simulink model "SYHW_Zscan"  (Simulink 8.1)
settings: Solver=ode5  SolverMode=SingleTasking  StartTime=0.0  StopTime=inf  FixedStep=Ts  RelTol=1e-3
PreLoadFcn:
  | Ts=20e-6;Ts_eHS=8e-7;parameters3;
PostLoadFcn:
  | Ts=20e-6;Ts_eHS=8e-7;parameters3;
InitFcn:
  | Ts=20e-6;Ts_eHS=8e-7;parameters3;
StartFcn:
  | Ts=20e-6;Ts_eHS=8e-7;parameters3;
undefined symbols (not defined in the file or in its folder): Fnom, opsimget, p, SW01
undefined symbols (not defined in the file): LmSI, LrSI, LsSI, RrSI, RsSI
libraries: rtlab x35, rtio_opalrt_common x13, efs_cpuhilios_crtl_lib x4, cpuhilios_lib x4, simulink x3, dspsigops x3, powerlib_extras x1, powerlib_meascontrol x1, rteventslib x1, cpuconverter_lib x1
(part 1 of 2)
settings Model: ARTEMISmethode_block_infos=$$__separator__$$  Creator=Administrator  LastModifiedBy=ncepri  BufferReuse=off
settings DataIOCC: LimitDataPoints=off  SaveFormat=StructureWithTime  SaveOutput=off  SignalLogging=off  DSMLogging=off  SaveTime=off
settings OptimizationCC: BlockReduction=off  OptimizeBlockIOStorage=off  BufferReuse=off  ExpressionFolding=off  LocalBlockOutputs=off
settings DebuggingCC: StrictBusMsg=None
settings GRTTargetCC: CodeReplacementLibrary=None  CPPClassGenCompliant=on
settings ConfigurationSet: Description=SimMechanics 2G

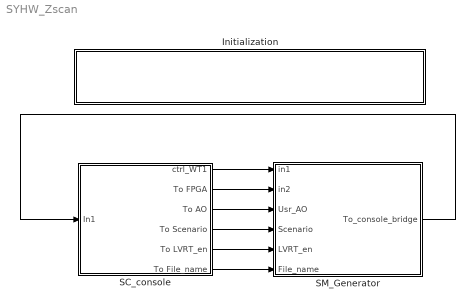
== system SYHW_Zscan ==
  Initialization : Subsystem  mask(Model Functions){InitFcnX=Ts=20e-6;Ts_eHS=8e-7;parameters3;, prel=on, posl=on, inif=on, strf=on}
      mask prompts: InitFcnX "Initialisation"; prel "Preload Function"; posl "PostLoad Function"; inif "InitFcn"; strf "StartFcn"
      mask init:
      | if prel==1
      | 	set_param(bdroot, 'PreLoadFcn', InitFcnX);
      | else
      | 	set_param(bdroot, 'PreLoadFcn', '');
      | end
      | if inif==1
      | 	set_param(bdroot, 'InitFcn', InitFcnX);
      | else
      | 	set_param(bdroot, 'InitFcn', '');
      | end
      | if strf==1
      | 	set_param(bdroot, 'StartFcn', InitFcnX);
      | else
      | 	set_param(bdroot, 'StartFcn', '');
      | end
      | if posl==1
      | 	set_param(bdroot, 'PostLoadFcn', InitFcnX);
      | else
      | 	set_param(bdroot, 'PostLoadFcn', '');
      | end
      | PLF = get_param(bdroot, 'PreLoadFcn');
      | IF = get_param(bdroot, 'InitFcn');
      | SF = get_param(bdroot, 'StartFcn');
      | 
      | 
      | pos = get_param(gcb, 'Position');
      | width = pos(3) - pos(1); height = pos(4) - pos(2);
      mask Display:
      | color('blue')
      | text(5, height*0.25, [ ...
      | upper(bdroot) '\n' ...
      | '- InitFcn. . . . . '  get_param(bdroot, 'InitFcn')  ...
      | ], ...
      | 'horizontalAlignment', 'left', 'verticalAlignment', 'middle') ;
      | text(60,height*0.6,'This is initilization control of the model');
  SC_console : Subsystem
  SM_Generator : Subsystem
  wires:
  SC_console/1(ctrl_WT1) -> SM_Generator/1(in1)
  SM_Generator/1(To_console_bridge) -> SC_console/1(In1)
  SC_console/2(To FPGA) -> SM_Generator/2(in2)
  SC_console/3(To AO) -> SM_Generator/3(Usr_AO)
  SC_console/4(To Scenario) -> SM_Generator/4(Scenario)
  SC_console/5(To LVRT_en) -> SM_Generator/5(LVRT_en)
  SC_console/6(To File_name) -> SM_Generator/6(File_name)

== system SYHW_Zscan/Initialization ==
  Model Info : simulink/Model-Wide Utilities/Model Info  InitialBlockCM=none  BlockCM=None  Frame=on  DisplayStringWithTags=|  HorizontalTextAlignment=Center  LeftAlignmentValue=0.5  SourceBlockDiagram=SYHW_Zscan  TagMaxNumber=20
      | - Version <<<1.0 >>>
      | 
      | - Description :
      | %<Description>
      | 
      | - Created by :     %<Creator>
      | - Creation date : %<Created>
      | - Modified by :    %<ModifiedBy>
      | - Last modif. :   2012.12.11

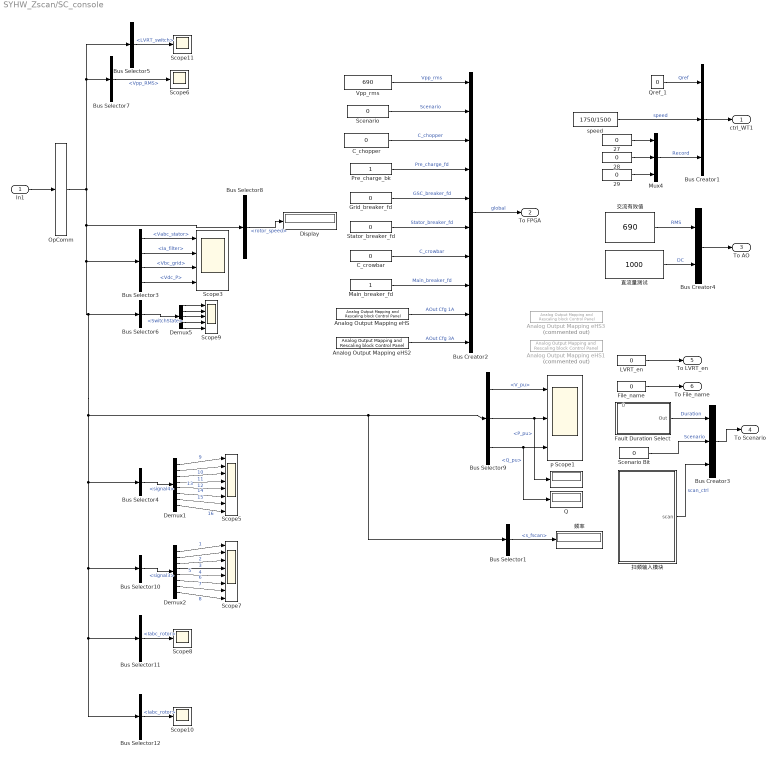
== system SYHW_Zscan/SC_console ==
  note: 0
  In1 : Inport
  " P" : Display
  " Q" : Display
  " 频率" : Display
  27 : Constant  Value=0
  28 : Constant  Value=0
  29 : Constant  Value=0
  Analog Output Mapping eHS : efs_cpuhilios_crtl_lib/Analog Output Mapping and  Rescaling block Control Panel  formFactor=Custom  SigNames={'eHS.Y01' 'eHS.Y02' 'eHS.Y03' 'eHS.Y04' 'eHS.Y05' 'eHS.Y06' 'eHS.Y07' 'eHS.Y08' 'eHS.Y09' 'eHS.Y10' 'eHS.Y11' 'eHS.Y12' 'eHS.Y13' 'eHS.Y14' 'eHS.Y15' 'eHS.Y16' 'eHS.Y17' 'eHS.Y18' 'eHS.Y19' 'eHS.Y20' 'eHS.Y21' 'eHS.Y22' 'eHS.Y23' 'eHS.Y24' 'eHS.Y25' 'eHS.Y26' 'eHS.Y27' 'eHS.Y28' 'eHS.Y29' 'eHS.Y30' 'eHS.Y31' 'eHS.Y32'}  NbUsrAOut=16  signalch0=eHS.Y22  gain0=10/1449  offset0=0  max0=10  min0=-10  signalch1=eHS.Y23  gain1=10/1449  offset1=0  max1=10  min1=-10  signalch2=eHS.Y24  gain2=10/1449  offset2=0  max2=10  min2=-10  signalch3=eHS.Y25  gain3=10/1449  offset3=0  max3=10  min3=-10  signalch4=eHS.Y26  gain4=10/1449  offset4=0  max4=10  min4=-10  signalch5=eHS.Y27  gain5=10/1449  offset5=0  max5=10  min5=-10  signalch6=eHS.Y07  gain6=10/1449  offset6=0  max6=10  min6=-10  signalch7=eHS.Y08  gain7=10/1449  offset7=0  max7=10  min7=-10  signalch8=eHS.Y09  gain8=10/1449  offset8=0  max8=10  min8=-10  signalch9=eHS.Y10  gain9=10/1449  offset9=0  max9=10  min9=-10  signalch10=eHS.Y11  gain10=10/1449  offset10=0  max10=10  min10=-10  signalch11=User16  gain11=0  offset11=0  max11=10  min11=0  signalch12=eHS.Y13  gain12=10/3200*1000/475  offset12=0  max12=10  min12=0  signalch13=User14  gain13=1/160  offset13=0  max13=10  min13=0  signalch14=User15  gain14=1/160  offset14=0  max14=10  min14=0  signalch15=User16  gain15=-10/1600  offset15=0  max15=10  min15=-10  signalch16=User1  gain16=0.0014  offset16=0  max16=5  min16=-5  signalch17=User2  gain17=0.0014  offset17=0  max17=5  min17=-5  signalch18=User3  gain18=0.0014  offset18=0  max18=5  min18=-5  signalch19=User4  gain19=0.00234  offset19=0  max19=5  min19=-5  signalch20=User5  gain20=0.00234  offset20=0  max20=5  min20=-5  signalch21=User6  gain21=0.00234  offset21=0  max21=5  min21=-5  signalch22=User7  gain22=0.00234  offset22=0  max22=5  min22=-5  signalch23=User7  gain23=0.00234  offset23=0  max23=5  min23=-5  signalch24=User9  gain24=0.00174  offset24=0  max24=3  min24=-3  signalch25=User10  gain25=0.000334  offset25=0  max25=3  min25=-3  signalch26=User11  gain26=0.000334  offset26=0  max26=3  min26=-3  signalch27=User12  gain27=0.000334  offset27=0  max27=3  min27=-3  signalch28=User13  gain28=1  offset28=0  max28=16  min28=-16  signalch29=User14  gain29=1  offset29=0  max29=16  min29=-16  signalch30=User15  gain30=1  offset30=0  max30=16  min30=-16  signalch31=User16  gain31=1  offset31=0  max31=16  min31=-16
      link override Display2: Decimation=12500
  Analog Output Mapping eHS1 : efs_cpuhilios_crtl_lib/Analog Output Mapping and  Rescaling block Control Panel  Commented=on  formFactor=Custom  SigNames={'eHS.Y01' 'eHS.Y02' 'eHS.Y03' 'eHS.Y04' 'eHS.Y05' 'eHS.Y06' 'eHS.Y07' 'eHS.Y08' 'eHS.Y09' 'eHS.Y10' 'eHS.Y11' 'eHS.Y12' 'eHS.Y13' 'eHS.Y14' 'eHS.Y15' 'eHS.Y16' 'eHS.Y17' 'eHS.Y18' 'eHS.Y19' 'eHS.Y20' 'eHS.Y21' 'eHS.Y22' 'eHS.Y23' 'eHS.Y24' 'eHS.Y25' 'eHS.Y26' 'eHS.Y27' 'eHS.Y28' 'eHS.Y29' 'eHS.Y30' 'eHS.Y31' 'eHS.Y32'}  NbUsrAOut=16  signalch0=eHS.Y01  gain0=1/240  offset0=0  max0=10  min0=-10  signalch1=eHS.Y02  gain1=1/240  offset1=0  max1=10  min1=-10  signalch2=eHS.Y03  gain2=1/240  offset2=0  max2=10  min2=-10  signalch3=eHS.Y08  gain3=1/722  offset3=0  max3=10  min3=-10  signalch4=eHS.Y09  gain4=1/722  offset4=0  max4=10  min4=-10  signalch5=eHS.Y10  gain5=1/240  offset5=0  max5=10  min5=-10  signalch6=eHS.Y21  gain6=1/240  offset6=0  max6=10  min6=-10  signalch7=eHS.Y22  gain7=1/240  offset7=0  max7=10  min7=-10  signalch8=eHS.Y23  gain8=10/1800*1  offset8=0  max8=10  min8=-10  signalch9=eHS.Y28  gain9=1/100  offset9=0  max9=10  min9=-10  signalch10=eHS.Y29  gain10=1/100  offset10=0  max10=10  min10=-10  signalch11=eHS.Y30  gain11=1/100  offset11=0  max11=14  min11=-14  signalch12=User13  gain12=4/300  offset12=0  max12=4  min12=0  signalch13=User14  gain13=-4/300  offset13=0  max13=5  min13=-5  signalch14=User15  gain14=-4/300  offset14=0  max14=5  min14=-5  signalch15=User16  gain15=4/300  offset15=0  max15=5  min15=0  signalch16=User1  gain16=4/300  offset16=0  max16=3  min16=-3  signalch17=User2  gain17=4/300  offset17=0  max17=4  min17=-4  signalch18=User3  gain18=4/300  offset18=0  max18=4  min18=-4  signalch19=User4  gain19=4/300  offset19=0  max19=4  min19=-4  signalch20=User5  gain20=0.0028427  offset20=0  max20=3  min20=-3  signalch21=User6  gain21=0.0028427  offset21=0  max21=3  min21=-3  signalch22=User7  gain22=0.0028427  offset22=0  max22=3  min22=-3  signalch23=User7  gain23=1  offset23=0  max23=3  min23=-3  signalch24=User9  gain24=1  offset24=0  max24=3  min24=-3  signalch25=User10  gain25=1  offset25=0  max25=16  min25=-16  signalch26=User11  gain26=1  offset26=0  max26=16  min26=-16  signalch27=User12  gain27=1  offset27=0  max27=16  min27=-16  signalch28=User13  gain28=1  offset28=0  max28=16  min28=-16  signalch29=User14  gain29=1  offset29=0  max29=16  min29=-16  signalch30=User15  gain30=1  offset30=0  max30=16  min30=-16  signalch31=User16  gain31=1  offset31=0  max31=16  min31=-16
      link override Display2: Decimation=12500
  Analog Output Mapping eHS2 : efs_cpuhilios_crtl_lib/Analog Output Mapping and  Rescaling block Control Panel  formFactor=Custom  SigNames={'eHS.Y01' 'eHS.Y02' 'eHS.Y03' 'eHS.Y04' 'eHS.Y05' 'eHS.Y06' 'eHS.Y07' 'eHS.Y08' 'eHS.Y09' 'eHS.Y10' 'eHS.Y11' 'eHS.Y12' 'eHS.Y13' 'eHS.Y14' 'eHS.Y15' 'eHS.Y16' 'eHS.Y17' 'eHS.Y18' 'eHS.Y19' 'eHS.Y20' 'eHS.Y21' 'eHS.Y22' 'eHS.Y23' 'eHS.Y24' 'eHS.Y25' 'eHS.Y26' 'eHS.Y27' 'eHS.Y28' 'eHS.Y29' 'eHS.Y30' 'eHS.Y31' 'eHS.Y32'}  NbUsrAOut=16  signalch0=eHS.Y14  gain0=-10/9000*500/330  offset0=0  max0=10  min0=-10  signalch1=eHS.Y15  gain1=-10/9000*500/330  offset1=0  max1=10  min1=-10  signalch2=eHS.Y16  gain2=-10/9000*500/330  offset2=0  max2=10  min2=-10  signalch3=eHS.Y17  gain3=10/10000  offset3=0  max3=10  min3=-10  signalch4=eHS.Y18  gain4=10/10000  offset4=0  max4=10  min4=-10  signalch5=eHS.Y19  gain5=-10/9000*500/330*398/473  offset5=0  max5=10  min5=-10  signalch6=eHS.Y20  gain6=-10/9000*500/330*398/473  offset6=0  max6=10  min6=-10  signalch7=eHS.Y21  gain7=-10/9000*500/330*398/473  offset7=0  max7=10  min7=-10  signalch8=eHS.Y23  gain8=0.00174*500/472*0  offset8=0  max8=3  min8=-3  signalch9=eHS.Y20  gain9=0.000251*353/348*1.315  offset9=0  max9=3  min9=-3  signalch10=eHS.Y21  gain10=0.000251*353/348*1.315  offset10=0  max10=3  min10=-3  signalch11=eHS.Y22  gain11=0.000251*353/348*1.315  offset11=0  max11=3  min11=-3  signalch12=eHS.Y11  gain12=0.00263*0.885*0.864  offset12=0  max12=4  min12=0  signalch13=User14  gain13=0.00263*0.885  offset13=0  max13=5  min13=-5  signalch14=User15  gain14=0.00263*0.885  offset14=0  max14=5  min14=-5  signalch15=User16  gain15=4/300  offset15=0  max15=5  min15=0  signalch16=User1  gain16=4/300  offset16=0  max16=3  min16=-3  signalch17=User2  gain17=4/300  offset17=0  max17=4  min17=-4  signalch18=User3  gain18=4/300  offset18=0  max18=4  min18=-4  signalch19=User4  gain19=4/300  offset19=0  max19=4  min19=-4  signalch20=User5  gain20=0.0028427  offset20=0  max20=3  min20=-3  signalch21=User6  gain21=0.0028427  offset21=0  max21=3  min21=-3  signalch22=User7  gain22=0.0028427  offset22=0  max22=3  min22=-3  signalch23=User7  gain23=1  offset23=0  max23=3  min23=-3  signalch24=User9  gain24=1  offset24=0  max24=3  min24=-3  signalch25=User10  gain25=1  offset25=0  max25=16  min25=-16  signalch26=User11  gain26=1  offset26=0  max26=16  min26=-16  signalch27=User12  gain27=1  offset27=0  max27=16  min27=-16  signalch28=User13  gain28=1  offset28=0  max28=16  min28=-16  signalch29=User14  gain29=1  offset29=0  max29=16  min29=-16  signalch30=User15  gain30=1  offset30=0  max30=16  min30=-16  signalch31=User16  gain31=1  offset31=0  max31=16  min31=-16
      link override Display2: Decimation=12500
  Analog Output Mapping eHS3 : efs_cpuhilios_crtl_lib/Analog Output Mapping and  Rescaling block Control Panel  Commented=on  formFactor=Custom  SigNames={'eHS.Y01' 'eHS.Y02' 'eHS.Y03' 'eHS.Y04' 'eHS.Y05' 'eHS.Y06' 'eHS.Y07' 'eHS.Y08' 'eHS.Y09' 'eHS.Y10' 'eHS.Y11' 'eHS.Y12' 'eHS.Y13' 'eHS.Y14' 'eHS.Y15' 'eHS.Y16' 'eHS.Y17' 'eHS.Y18' 'eHS.Y19' 'eHS.Y20' 'eHS.Y21' 'eHS.Y22' 'eHS.Y23' 'eHS.Y24' 'eHS.Y25' 'eHS.Y26' 'eHS.Y27' 'eHS.Y28' 'eHS.Y29' 'eHS.Y30' 'eHS.Y31' 'eHS.Y32'}  NbUsrAOut=16  signalch0=eHS.Y01  gain0=1/120  offset0=0  max0=8  min0=-8  signalch1=eHS.Y02  gain1=1/120  offset1=0  max1=8  min1=-8  signalch2=eHS.Y03  gain2=1/120  offset2=0  max2=8  min2=-8  signalch3=eHS.Y08  gain3=1/120  offset3=0  max3=10  min3=-10  signalch4=eHS.Y09  gain4=1/120  offset4=0  max4=10  min4=-10  signalch5=eHS.Y10  gain5=1/120  offset5=0  max5=10  min5=-10  signalch6=eHS.Y21  gain6=1/120  offset6=0  max6=10  min6=-10  signalch7=eHS.Y22  gain7=1/120  offset7=0  max7=10  min7=-10  signalch8=eHS.Y23  gain8=1/120  offset8=0  max8=10  min8=-10  signalch9=eHS.Y28  gain9=1/153  offset9=0  max9=10  min9=-10  signalch10=eHS.Y29  gain10=1/153  offset10=0  max10=10  min10=-10  signalch11=eHS.Y30  gain11=1/320  offset11=0  max11=10  min11=0  signalch12=User13  gain12=1/160  offset12=0  max12=10  min12=0  signalch13=User14  gain13=1/160  offset13=0  max13=10  min13=0  signalch14=User15  gain14=1/160  offset14=0  max14=10  min14=0  signalch15=User16  gain15=-10/1600  offset15=0  max15=10  min15=-10  signalch16=User1  gain16=1  offset16=0  max16=3  min16=-3  signalch17=User2  gain17=4/300  offset17=0  max17=4  min17=-4  signalch18=User3  gain18=4/300  offset18=0  max18=4  min18=-4  signalch19=User4  gain19=4/300  offset19=0  max19=4  min19=-4  signalch20=User5  gain20=0.0028427  offset20=0  max20=3  min20=-3  signalch21=User6  gain21=0.0028427  offset21=0  max21=3  min21=-3  signalch22=User7  gain22=0.0028427  offset22=0  max22=3  min22=-3  signalch23=User7  gain23=1  offset23=0  max23=3  min23=-3  signalch24=User9  gain24=1  offset24=0  max24=3  min24=-3  signalch25=User10  gain25=1  offset25=0  max25=16  min25=-16  signalch26=User11  gain26=1  offset26=0  max26=16  min26=-16  signalch27=User12  gain27=1  offset27=0  max27=16  min27=-16  signalch28=User13  gain28=1  offset28=0  max28=16  min28=-16  signalch29=User14  gain29=1  offset29=0  max29=16  min29=-16  signalch30=User15  gain30=1  offset30=0  max30=16  min30=-16  signalch31=User16  gain31=1  offset31=0  max31=16  min31=-16
      link override Display2: Decimation=12500
  Bus Creator1 : BusCreator  Inputs=3
  Bus Creator2 : BusCreator  Inputs=10
  Bus Creator3 : BusCreator  Inputs=3
  Bus Creator4 : BusCreator  Inputs=2
  Bus Selector1 : BusSelector  OutputSignals=s_fscan
  Bus Selector10 : BusSelector  OutputSignals=DI_state.signal3
  Bus Selector11 : BusSelector  OutputSignals=Iabc_rotor
  Bus Selector12 : BusSelector  OutputSignals=Iabc_rotor
  Bus Selector3 : BusSelector  OutputSignals=Vabc_stator,Ia_filter,Vbc_grid,Vdc_P
  Bus Selector4 : BusSelector  OutputSignals=DI_state.signal4
  Bus Selector5 : BusSelector  OutputSignals=LVRT_switch
  Bus Selector6 : BusSelector  OutputSignals=SwitchState
  Bus Selector7 : BusSelector  OutputSignals=Vpp_RMS
  Bus Selector8 : BusSelector  OutputSignals=rotor_speed
  Bus Selector9 : BusSelector  OutputSignals=pu_meas_690.V_pu,pu_meas_690.P_pu,pu_meas_690.Q_pu
  C_chopper : Constant  Value=0
  C_crowbar : Constant  Value=0
  Demux1 : Demux  Outputs=8
  Demux2 : Demux  Outputs=8
  Demux5 : Demux  Outputs=5
  Display : Display
  Fault Duration Select : Subsystem  mask{var_dur=20% - 0.625 sec}
      mask prompts: var_dur "Duration"
      mask TypeOptions var_dur: 20% - 0.625 sec | 35% - 0.92 sec | 50% - 1.214 sec | 75% - 1.705 sec | 90% - 2.0 sec | 130% - 0.5 sec | 125% - 1.0 sec | 120% - 10 sec
      mask Display:
      | fault_vector = {'20%', '35%', '50%', '75%', '90%', '130%', '125%', '120%'};
      | dur_vector = [0.625, 0.92, 1.214, 1.705, 2.0, 0.5, 1.0, 10.0];
      | text(10, 25, strcat(fault_vector{var_dur}, ' - ', num2str(dur_vector(var_dur)), ' sec'))
  File_name : Constant  Value=0
  Grid_breaker_fd : Constant  Value=0
  LVRT_en : Constant  Value=0
  Main_breaker_fd : Constant
  Mux4 : Mux  Inputs=3
  OpComm : rtlab/OpComm  nbport=1  groupe_acq=1  subsys_rate=0  st=0  Synchronization=off  Interpolation=on  Threshold=1.0  Missed_Data=off  Sim_Time=off  Samples=off  dynSigOut=off  from_console=0  warning_done=off  writeOpCommFile=off  Offset=off
  Pre_charge_bk : Constant
  Qref_1 : Constant  Value=0
  Scenario : Constant  Value=0
  Scenario Bit : Constant  Value=0
  Scope1 : Scope  NumInputPorts=3
      settings: YMin=-0.1~-0.1~-1.2  YMax=1.4~1.2~1.2
  Scope{6,8,10..11} (4 alike) : Scope
      Scope10 settings: YMin=-1  YMax=1  SaveName=ScopeData10
      Scope11 settings: SaveName=ScopeData11
      Scope6 settings: SaveName=ScopeData6
      Scope8 settings: YMin=-1  YMax=1  SaveName=ScopeData9
  Scope3 : Scope  NumInputPorts=4
      settings: YMin=-5~-5~-5~-5  YMax=5~5~5~5  SaveName=ScopeData3
  Scope5 : Scope  NumInputPorts=8
      settings: YMin=-5~-5~-5~-5~-5~-5~-5~-5  YMax=5~5~5~5~5~5~5~5  SaveName=ScopeData4
  Scope7 : Scope  NumInputPorts=8
      settings: YMin=-5~-5~-5~-5~-5~-5~-5~-5  YMax=5~5~5~5~5~5~5~5  SaveName=ScopeData5
  Scope9 : Scope  NumInputPorts=5
      settings: YMin=-5~-5~-5~-5~-5  YMax=5~5~5~5~5  SaveName=ScopeData8
  Stator_breaker_fd : Constant  Value=0
  Vpp_rms : Constant  Value=690
  speed : Constant  Value=1750/1500
  交流有效值 : Constant  Value=690
  扫频输入模块 : Subsystem  mask{ScanStart=0, DisRatio1=0.005, DisRatio2=0.02, fileNum=0}
      mask prompts: ScanStart "1：启动扫频，0：停止扫频"; DisRatio1 "1-20Hz扰动百分比"; DisRatio2 "20Hz之后扰动百分比"; fileNum "文件编号"
  直流量测试 : Constant  Value=1000
  ctrl_WT1 : Outport
  To FPGA : Outport  Port=2
  To AO : Outport  Port=3
  To Scenario : Outport  Port=4
  To LVRT_en : Outport  Port=5
  To File_name : Outport  Port=6
  wires:
  In1/1 -> OpComm/1
  Bus Creator2/1 -> To FPGA/1  "global"
  Pre_charge_bk/1 -> Bus Creator2/4  "Pre_charge_fd"
  Grid_breaker_fd/1 -> Bus Creator2/5  "GSC_breaker_fd"
  Stator_breaker_fd/1 -> Bus Creator2/6  "Stator_breaker_fd"
  Bus Creator4/1 -> To AO/1
  Bus Creator1/1 -> ctrl_WT1/1
  27/1 -> Mux4/1
  28/1 -> Mux4/2
  29/1 -> Mux4/3
  Mux4/1 -> Bus Creator1/3  "Record"
  Qref_1/1 -> Bus Creator1/1  "Qref"
  speed/1 -> Bus Creator1/2  "speed"
  Analog Output Mapping eHS2/1 -> Bus Creator2/10  "AOut Cfg 3A"
  Analog Output Mapping eHS/1 -> Bus Creator2/9  "AOut Cfg 1A"
  C_crowbar/1 -> Bus Creator2/7  "C_crowbar"
  Main_breaker_fd/1 -> Bus Creator2/8  "Main_breaker_fd"
  Vpp_rms/1 -> Bus Creator2/1  "Vpp_rms"
  Scenario/1 -> Bus Creator2/2  "Scenario"
  C_chopper/1 -> Bus Creator2/3  "C_chopper"
  LVRT_en/1 -> To LVRT_en/1
  Bus Selector5/1 -> Scope11/1  "<LVRT_switch>"
  Bus Selector3/3 -> Scope3/3  "<Vbc_grid>"
  Bus Selector3/4 -> Scope3/4  "<Vdc_P>"
  Bus Selector3/2 -> Scope3/2  "<Ia_filter>"
  Bus Selector3/1 -> Scope3/1  "<Vabc_stator>"
  Bus Selector6/1 -> Demux5/1  "<SwitchState>"
  Demux5/3 -> Scope9/3
  Demux5/1 -> Scope9/1
  Demux5/2 -> Scope9/2
  Demux5/4 -> Scope9/4
  Demux5/5 -> Scope9/5
  Bus Selector7/1 -> Scope6/1  "<Vpp_RMS>"
  Bus Selector8/1 -> Display/1  "<rotor_speed>"
  Bus Selector9/1 -> Scope1/1  "<V_pu>"
  File_name/1 -> To File_name/1
  Demux1/3 -> Scope5/3  "11"
  Demux1/1 -> Scope5/1  "9"
  Demux1/2 -> Scope5/2  "10"
  Demux1/4 -> Scope5/4  "12"
  Demux1/5 -> Scope5/5  "13"
  Bus Selector4/1 -> Demux1/1  "<signal4>"
  Demux1/6 -> Scope5/6  "14"
  Demux1/7 -> Scope5/7  "15"
  Demux1/8 -> Scope5/8  "16"
  Demux2/3 -> Scope7/3  "3"
  Demux2/1 -> Scope7/1  "1"
  Demux2/2 -> Scope7/2  "2"
  Demux2/4 -> Scope7/4  "4"
  Demux2/5 -> Scope7/5  "5"
  Bus Selector10/1 -> Demux2/1  "<signal3>"
  Demux2/6 -> Scope7/6  "6"
  Demux2/7 -> Scope7/7  "7"
  Demux2/8 -> Scope7/8  "8"
  Bus Selector11/1 -> Scope8/1  "<Iabc_rotor>"
  Bus Selector12/1 -> Scope10/1  "<Iabc_rotor>"
  Bus Creator3/1 -> To Scenario/1
  Fault Duration Select/1(Out) -> Bus Creator3/1  "Duration"
  Scenario Bit/1 -> Bus Creator3/2  "Scenario"
  交流有效值/1 -> Bus Creator4/1  "RMS"
  直流量测试/1 -> Bus Creator4/2  "DC"
  OpComm/1 -> Bus Selector12/1, Bus Selector11/1, Bus Selector10/1, Bus Selector4/1, Bus Selector1/1, Bus Selector9/1, Bus Selector6/1, Bus Selector3/1, Bus Selector8/1, Bus Selector7/1, Bus Selector5/1
  Bus Selector1/1 -> " 频率"/1  "<s_fscan>"
  扫频输入模块/1(scan) -> Bus Creator3/3  "scan_ctrl"
  Bus Selector9/2 -> " P"/1, Scope1/2  "<P_pu>"
  Bus Selector9/3 -> " Q"/1, Scope1/3  "<Q_pu>"

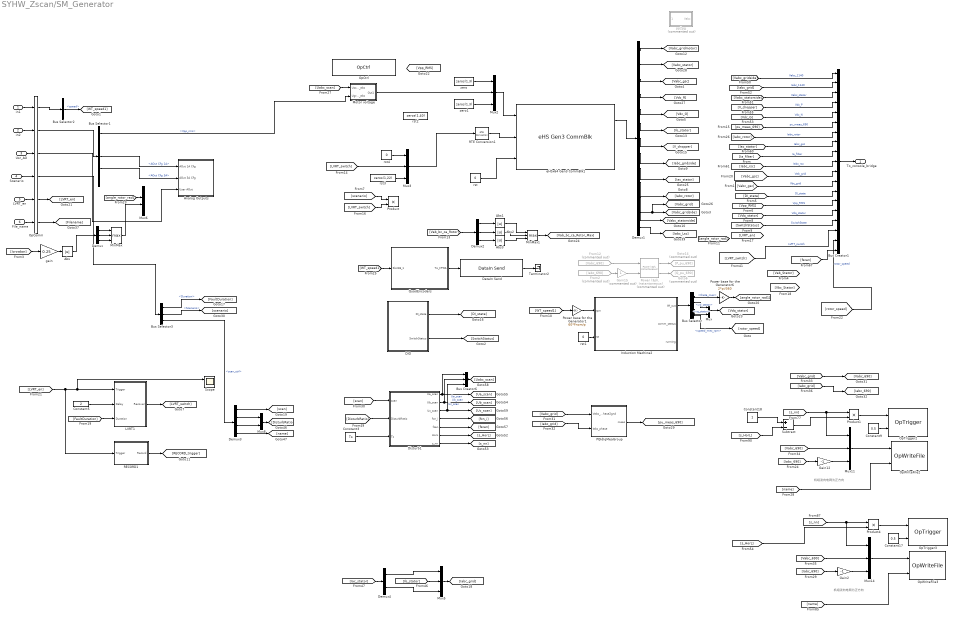
== system SYHW_Zscan/SM_Generator ==
  note: 机组流向电网为正方向
  note: 机组流向电网为正方向
  in1 : Inport
  in2 : Inport  Port=2
  Usr_AO : Inport  Port=3
  Scenario : Inport  Port=4
  LVRT_en : Inport  Port=5
  File_name : Inport  Port=6
  Abs{,1..3} (4 alike) : Abs
  Analog Outputs : Subsystem
  Bus Creator1 : BusCreator  Inputs=19
  Bus Creator6 : BusCreator  Inputs=3
  Bus Selector : BusSelector  OutputSignals=theta_mec,vd_stator,vq_stator,speed_mec_rpm
  Bus Selector1 : BusSelector  OutputSignals=Vpp_rms,Scenario,AOut Cfg 1A,AOut Cfg 3A,C_chopper
  Bus Selector2 : BusSelector  OutputSignals=speed
  Bus Selector3 : BusSelector  OutputSignals=Duration,Scenario,scan_ctrl
  Constant17 : Constant  Value=0.5
  Constant18 : Constant
  Constant3 : Constant  Value=Ts
  Constant5 : Constant  Value=2
  Constant9 : Constant  Value=0.5
  DIO : Subsystem
  DataIn Send : rtio_opalrt_common/DataIn Send  CtrlName='eHS Ctrl'  FcnNos=30  width=1  portType=uint32  checkVersion=off  expectedId=0  expectedVersion=0  opComp=>=
      settings: AttributesFormatString=%<CtrlName>
  Demux : Demux  Outputs=3
  Demux1 : Demux  Outputs=[3 3 3 1 1 1 1 3 2 3 3 3 3]
  Demux2 : Demux  Outputs=3
  Demux3 : Demux
  Demux4 : Demux  Outputs=2
  Disturb1 : Subsystem  mask{UofPCC=690}
      mask prompts: UofPCC "并网点电压（V)"
      settings: ErrorFcn=扫频步长
  From12 : From  Commented=on  GotoTag=Vabc_690
      settings: CloseFcn=tagdialog Close
  From2 : From  Commented=on  GotoTag=Iabc_690
      settings: CloseFcn=tagdialog Close
  Gain12 : Gain  Gain=-1  SampleTime=Ts
  Gain15 : Gain  Commented=on
  Gain2 : Gain  Gain=-1  SampleTime=Ts
  Goto14 : Goto  Commented=on  GotoTag=P_pu_690
  Goto6 : Goto  Commented=on  GotoTag=Q_pu_690
  Induction Machine2 : Subsystem  AncestorBlock=cpumachines_lib/Induction Machine  mask(eFPGAsim Induction Machine){param_in=off, Lls=LsSI, Rs=RsSI, Llr=LrSI, Rr=RrSI, Lm=LmSI, pp=p, fixrefangle=0, show_vforce=off, dt=Ts_eHS, CtrlName='eHS Ctrl', period=5e-9, PortNb1=27, PortNb2=22, PortNb3=3, PortNb4=23}
      mask prompts: param_in "Parameters as inports of the block"; Lls "Stator Inductance:"; Rs "Stator Resistance:"; Llr "Rotor Inductance:"; Rr "Rotor Resistance:"; Lm "Mutual Inductance:"; pp "Pole Pairs:"; fixrefangle "Fix referential angle:"; show_vforce "Show Rotor/Stator Voltages override ports"; dt "Solver Time Step: [sec]"; CtrlName "Hardware Controller Name (OpCtrl)"; period "FPGA Clock period: [sec]"; PortNb1 "Configuration Port Number: Configuration file (LoadIn)"; PortNb2 "Configuration Port Number: Speed, Parameters, Forces Voltage (DataIn Send)"; PortNb3 "Configuration Port Number: Outputs (DataOut Recv)"; PortNb4 "Configuration Port Number: MTX (DataIn Send)"
      mask help: The Induction machine block implements the driver of the FPGA-based 3phase Inducation Machine (IM) model. The settings of this parameter panel are transformed into the control signals of the FPGA-based machine.
      mask init:
      | efsInductionMotorCb(gcb,'ParamIn');
      | efsInductionMotorCb(gcb,'ShowVforce');
      | efsInductionMotorCb(gcb,'MaskInitFcn', Lls, Rs, Llr, Rr, Lm , pp, fixrefangle, dt, period)
      settings: PreDeleteFcn=efsInductionMotorCb(gcb,'PreDeleteFcn')
      mask Help: web(['file:///' getenv('EFPGASIM_ROOT') '/Docs/html/eFPGAsim/efs_cpuIM.html']);
  LVRT1 : Subsystem  mask{delay=2, duration=0.5}
      mask prompts: delay "故障延时（s）"; duration "故障时长（s）"
  MinMax : MinMax  Function=max  Inputs=3
  MinMax1 : MinMax  Function=max  Inputs=3
  Motor voltage : Subsystem
  Mux : Mux  Inputs=2
  Mux{3,5,11,14} (4 alike) : Mux  Inputs=3
  Mux2 : Mux  Inputs=[3 3 3]
  Mux6 : Mux
  Mux8 : Mux  Inputs=2
  OpComm : rtlab/OpComm  nbport=6  groupe_acq=1  subsys_rate=0  st=0  Synchronization=on  Interpolation=on  Threshold=1.0  Missed_Data=off  Sim_Time=off  Samples=off  dynSigOut=off  from_console=1  warning_done=off  writeOpCommFile=off  Offset=off
  OpCtrl : rtio_opalrt_common/OpCtrl  CtrlName='eHS Ctrl'  boardid=0  BitstreamFilename=VC707_2-EX-0001-2_3_6_104-eHSgen3_2PMSM_efs143_IOs_encoder-05-01.bin  numconfig=-1  mode=Master  externalClock=off  decimRtsi=0  calibIO=off  SampleTime=0  loadinport=-1  BoardType=VC707  SecondaryPresent=off  sync_type=Audio
  OpTrigger2 : rtlab/DataLogging/OpTrigger  Trig_Type=TRIGGER SIGNAL >= TRIGGER LEVEL  Trig_Offset=0  Acq_Group=27
  OpTrigger3 : rtlab/DataLogging/OpTrigger  Trig_Type=TRIGGER SIGNAL >= TRIGGER LEVEL  Trig_Offset=0  Acq_Group=28
  OpWriteFile2 : rtlab/DataLogging/OpWriteFile  Static_File=off  varname=Lscan  Filename=Lfile.mat  rtpath='./'  nrtpath='.\'  Acq_Group=27  file_size=1200000000*2.5  write_offline=off  Sim_Mode=off  Nb_Samples=10000  Buffer_size=floor(1e-4/Ts)*10000*8*8*1.2
      settings: Decimation=5
  OpWriteFile3 : rtlab/DataLogging/OpWriteFile  Static_File=off  varname=Hscan  Filename=Hfile.mat  rtpath='./'  nrtpath='.\'  Acq_Group=28  file_size=1200000000*2.5  write_offline=off  Sim_Mode=off  Nb_Samples=floor(1e-4/Ts)*10000  Buffer_size=floor(1e-4/Ts)*10000*8*8*1.2
  PQIdIqMeaGroup : Subsystem  mask{var_pnom=6.25e6, var_vline_rms=690, var_ts=Ts}
      mask prompts: var_pnom "Pnom"; var_vline_rms "Line voltage rms"; var_ts "Sample Time"
      mask help: 正序量计算模块封装
      mask Help: by Yamin
  "Power (3ph, Instantaneous)" : powerlib_meascontrol/Measurements/Power (3ph, Instantaneous)  Commented=on
  Power base for the Generator1 : Gain  Gain=60*Fnom/p  SaturateOnIntegerOverflow=on  OutDataTypeStr=Inherit: Same as input  ParamDataTypeStr=Inherit: Same as input
  Power base for the Generator6 : Gain  Gain=2*pi/360  SaturateOnIntegerOverflow=on  OutDataTypeStr=Inherit: Same as input  ParamDataTypeStr=Inherit: Same as input
  Product : Product
  Product1 : Product
  Product4 : Product
  QuadEncoders : Subsystem
  RECORD1 : Subsystem  mask{rec_time=20}
      mask prompts: rec_time "录波时长（s）"
  RTE Conversion1 : rteventslib/Signal Attributes/RTE Conversion  inputdatatype=Double  outputdatatype=RTE Boolean  compensation=Enabled  nbMaxEvents=10  sampleTime=Ts
  Scope : Scope  NumInputPorts=2
      settings: YMin=0.95~-1  YMax=1.05~1  SaveName=ScopeData13
  Subtract : Sum  Inputs=+-
  Terminator2 : Terminator
  eHSx64 Gen3 CommBlk1 : cpuconverter_lib/eHS Gen3 CommBlk  GenMat=off  solver_size=x64  circuit_mtx1=netlist_SY_HW_6p25MW_Zscan  Ts_eHS_1_explicit=off  Ts_eHS_1=5.75e-07  SimeHS1=off  ShowAdv1=on  gs1="0.8  %[0.8*ones(1,22) 0.25*0.25*0.25*0.8*ones(1,3) 0.8*ones(1,9)]"  v_init1=zeros(1,24)  i_init1=zeros(1,24)  netlist_name=netlist_SY_HW_6p25MW_Zscan.mdl  ts_min=5.75e-07  nb_u=9  input_names=U01 | U02 | U03 | U04 Va | U05 Vb | U06 Vc | U07 | U08 | U09  nb_sw=28  switches_names=Diode | Diode1 | Diode2 | Diode3 | Diode4 | Diode5 | SW01-06 GSC_01 | SW01-06 GSC_02 | SW01-06 GSC_03 | SW01-06 GSC_04 | SW01-06 GSC_05 | SW01-06 GSC_06 | SW07-12 RSC_01 | SW07-12 RSC_02 | SW07-12 RSC_03 | SW07-12 RSC_04 | SW07-12 RSC_05 | SW07-12 RSC_06 | SW14 | SW15-17/Breaker A | SW15-17/Breaker B | SW15-17/Breaker C | SW18-20/Breaker A | SW18-20/Breaker B | SW18-20/Breaker C | SW21-SW23/Breaker A | SW21-SW23/Breaker B | SW21-SW23/Breaker C  nb_y=30  output_names=Y01 | Y02 | Y03 | Y04 | Y05 | Y06 | Y07 | Y08 | Y09 | Y10 | Y11 | Y12 | Y13 | Y14 | Y15 | Y16 | Y17 | Y18 | Y19 | Y20 | Y21 | Y22 | Y23 | Y24 | Y25 | Y26 | Y27 | Y28 | Y29 | Y30  nb_nsd=34  Input_config1_popup=Independent setting for each element  input_config_1=[ 2 0 ; 2 1 ; 2 2 ; 0 3 ; 0 4 ; 0 5 ; 2 6 ; 2 7 ; 2 8 ]  input_nb_auto=on  input_nb=9  UseSWG=off  SWGPortNbs=3  Pulse_ctrl1_popup=Independent setting for each element  GateCtrlSelPanel=off  Pulse_ctrl1=[ 0 0 ; 0 1 ; 0 2 ; 0 3 ; 0 4 ; 0 5 ; 2 0 ; 2 1 ; 2 2 ; 2 3 ; 2 4 ; 2 5 ; 2 6 ; 2 7 ; 2 8 ; 2 9 ; 2 10 ; 2 11 ; 2 13 ; 2 32 ; 2 32 ; 2 32 ; 2 33 ; 2 33 ; 2 33 ; 2 34 ; 2 34 ; 2 34 ]  Polarity1_popup=Independent setting for each element  Polarity1=[ 0 0 0 0 0 0 0 0 0 0 0 0 0 0 0 0 0 0 0 1 1 1 1 1 1 1 1 1 ]  pulse_nb=24  rte_pulse_nb=SW01-24  nb_event=4  static_pulse=none  scn_en=off  xls_file=LVRT_3ph.xls  scn_cmd=do nothing  xls_page=1  nscn_max=8  nscn_used=1  scn_log_en=on  CtrlName='eHS Ctrl'  Ts=Ts  set_comm_port=on  PortNbs=[1 2 1 2:1:2+8 1]  isSwitchesLossesBlockPresent=on  switchesLossesBlockName=Thermal losses
      settings: AttributesFormatString=%<CtrlName>
  gain : Gain  Gain=0.25  SaturateOnIntegerOverflow=on  OutDataTypeStr=Inherit: Same as input  ParamDataTypeStr=Inherit: Same as input
  pp2pg : Subsystem  Commented=on
  rst : Constant  Value=0
  rst1 : Constant  Value=0
  rst2 : Constant  Value=zeros(1,40)
  rst3 : Constant  Value=zeros(1,22)
  rst4 : Constant  Value=0
  zero : Constant  Value=zeros(1,3)
  zero1 : Constant  Value=zeros(1,3)
  To_console_bridge : Outport
  wires:
  in1/1 -> OpComm/1
  OpComm/1 -> Bus Selector2/1
  zero/1 -> Mux2/1
  Bus Selector/1 -> Power base for the Generator6/1  "<theta_mec>"
  Power base for the Generator6/1 -> [angle_rotor_rad1]
  Bus Selector2/1 -> [WT_speed1]  "<speed>"
  in2/1 -> OpComm/2
  OpComm/2 -> Bus Selector1/1
  Bus Selector1/3 -> Analog Outputs/1(AOut 1A Cfg)  "<AOut Cfg 1A>"
  Bus Selector1/4 -> Analog Outputs/2(AOut 3A Cfg)  "<AOut Cfg 3A>"
  Usr_AO/1 -> OpComm/3
  [angle_rotor_rad1] -> Mux6/2
  OpComm/3 -> Analog Outputs/3(User AOut)
  [Icrowbar] -> gain/1
  gain/1 -> Abs/1
  Abs/1 -> Demux/1
  Demux/1 -> MinMax/1
  Demux/2 -> MinMax/2
  Demux/3 -> MinMax/3
  MinMax/1 -> Mux6/3
  [WT_speed1] -> QuadEncoders/1(Slot1B_1)
  QuadEncoders/1(To_FPGA) -> DataIn Send/1
  DataIn Send/1 -> Terminator2/1
  From2/1 -> Gain15/1
  Bus Creator1/1 -> To_console_bridge/1
  [Vabc_gridside] -> Bus Creator1/1  "Vabc_1140"
  [Iabc_grid] -> Bus Creator1/2  "Iabc_1140"
  [V_chopper] -> Bus Creator1/4  "Vdc_P"
  [Vdc_G] -> Bus Creator1/5  "Vdc_N"
  [Iabc_rsc] -> Bus Creator1/10  "Iabc_rsc"
  [Iac_stator] -> Bus Creator1/8  "Iabc_gsc"
  [Iabc_rotor] -> Bus Creator1/7  "Iabc_rotor"
  [Ia_filter] -> Bus Creator1/9  "Ia_filter"
  [Vabc_gsc] -> Bus Creator1/12  "Vbc_grid"
  Gain15/1 -> "Power (3ph, Instantaneous)"/2
  eHSx64 Gen3 CommBlk1/1 -> Demux1/1
  Demux1/3 -> [Vabc_gsc]
  Demux1/4 -> [Vdc_R]
  Demux1/5 -> [Vdc_G]
  Demux1/6 -> [Ib_stator]
  Demux1/7 -> [V_chopper]
  Demux1/8 -> [Iabc_gridside]
  Demux1/9 -> [Iac_stator]
  Demux1/10 -> [Iabc_rotor]
  Scenario/1 -> OpComm/4
  LVRT_en/1 -> OpComm/5
  OpComm/5 -> [LVRT_en]
  [DI_state] -> Bus Creator1/13  "DI_state"
  DIO/1(DI_state) -> [DI_state]
  [Vpp_RMS] -> Bus Creator1/14  "Vpp_RMS"
  Bus Selector/2 -> Mux/1  "<vd_stator>"
  Bus Selector/3 -> Mux/2  "<vq_stator>"
  Mux/1 -> [Vdq_stator]
  [Vdq_stator] -> Bus Creator1/15  "Vdq_stator"
  [WT_speed1] -> Power base for the Generator1/1
  Demux1/1 -> [Vabc_gridmotor]
  Demux1/2 -> [Vabc_stator]
  Induction Machine2/1(IM_out) -> Bus Selector/1
  Power base for the Generator1/1 -> Induction Machine2/1(rpm)
  rst1/1 -> Induction Machine2/2(rst)
  [Vabc_statorside] -> Bus Creator1/3  "Vabc_stator"
  [SwitchStatus] -> Bus Creator1/16  "SwitchState"
  [Vab_bc_ca_Rotor] -> Demux2/1
  Demux2/1 -> Abs1/1
  Demux2/2 -> Abs2/1
  Demux2/3 -> Abs3/1
  Abs1/1 -> MinMax1/1
  Abs2/1 -> MinMax1/2
  Abs3/1 -> MinMax1/3
  MinMax1/1 -> [Vab_bc_ca_Rotor_Max]
  DIO/2(SwitchStatus) -> [SwitchStatus]
  From12/1 -> "Power (3ph, Instantaneous)"/1
  "Power (3ph, Instantaneous)"/1 -> Goto14/1
  "Power (3ph, Instantaneous)"/2 -> Goto6/1
  [LVRT_switch] -> Bus Creator1/17  "LVRT_switch"
  rst3/1 -> Mux3/3
  rst4/1 -> Mux3/1
  [LVRT_switch] -> Mux3/2
  RECORD1/1(Record) -> [RECORD_trigger]
  [LVRT_en] -> LVRT1/1(Trigger), Scope/1, RECORD1/1(Trigger)
  Constant5/1 -> LVRT1/2(Delay)
  [FaultDuration] -> LVRT1/3(Duration)
  [rotor_speed] -> Bus Creator1/18  "rotor_speed"
  Mux3/1 -> RTE Conversion1/1
  zero1/1 -> Mux2/3
  [Vabc_gsc] -> Bus Creator1/11  "Vab_grid"
  Bus Selector/4 -> [rotor_speed]  "<speed_mec_rpm>"
  File_name/1 -> OpComm/6
  OpComm/6 -> [Filename]
  Demux1/11 -> [Vabc_grid], [Vabc_gridside]
  Demux1/12 -> [Vabc_statorside]
  [Iac_stator] -> Demux4/1
  [Ib_stator] -> Mux5/2
  Demux4/1 -> Mux5/1
  Demux4/2 -> Mux5/3
  Mux5/1 -> [Iabc_grid]
  Demux1/13 -> [Iabc_Lsc]
  LVRT1/1(Recover) -> [LVRT_switch]
  Mux2/1 -> eHSx64 Gen3 CommBlk1/1
  RTE Conversion1/1 -> eHSx64 Gen3 CommBlk1/2
  rst/1 -> eHSx64 Gen3 CommBlk1/3
  PQIdIqMeaGroup/1(meas) -> [pu_meas_690]
  [Vabc_grid] -> PQIdIqMeaGroup/1(Vabc_phase2gnd)
  [Iabc_grid] -> PQIdIqMeaGroup/2(Iabc_phase)
  [pu_meas_690] -> Bus Creator1/6  "pu_meas_690"
  OpComm/4 -> Bus Selector3/1
  Bus Selector3/1 -> [FaultDuration]  "<Duration>"
  [scenario] -> Product/1
  [LVRT_switch] -> Product/2
  Bus Selector1/1 -> Motor voltage/2(Ugrid_abc)  "<Vpp_rms>"
  [Uabc_scan] -> Motor voltage/1(Uscan_abc)
  Motor voltage/1(Out1) -> Mux2/2
  Disturb1/5(fsan) -> [fscan]
  Disturb1/4(fcn_i) -> [fcn_i]
  [scan] -> Disturb1/1(scan)
  Disturb1/1(Ua_scan) -> [Ua_scan], Bus Creator6/1  "Ua_scan"
  Disturb1/2(Ub_scan) -> Bus Creator6/2, [Ub_scan]  "Ub_scan"
  Disturb1/3(Uc_scan) -> Bus Creator6/3, [Uc_scan]  "Uc_scan"
  Bus Creator6/1 -> [Uabc_scan]
  [DisturbRatio] -> Disturb1/2(DisturbRatio)
  Constant3/1 -> Disturb1/3(Ts)
  Disturb1/6(HorL) -> [s_HorL]
  Disturb1/7("s_nn ") -> [s_nn]
  Demux3/1 -> [scan]
  Mux8/1 -> [DisturbRatio]
  Demux3/2 -> Mux8/1
  Demux3/3 -> Mux8/2
  Demux3/4 -> [name]
  Bus Selector3/2 -> [scenario]  "<Scenario>"
  Bus Selector3/3 -> Demux3/1  "<scan_ctrl>"
  Constant9/1 -> OpTrigger2/2
  Product1/1 -> OpTrigger2/1
  [s_nn] -> Product1/1, Mux11/1
  Subtract/1 -> Product1/2
  Mux11/1 -> OpWriteFile2/1
  [Iabc_690] -> Gain12/1
  [Vabc_690] -> Mux11/2
  Gain12/1 -> Mux11/3
  [name] -> OpWriteFile2/2
  Constant17/1 -> OpTrigger3/2
  Product4/1 -> OpTrigger3/1
  [s_nn] -> Product4/1, Mux14/1
  Mux14/1 -> OpWriteFile3/1
  [Iabc_690] -> Gain2/1
  [Vabc_690] -> Mux14/2
  Gain2/1 -> Mux14/3
  [name] -> OpWriteFile3/2
  Constant18/1 -> Subtract/1
  [s_HorL] -> Product4/2
  [s_HorL] -> Subtract/2
  [Vabc_grid] -> [Vabc_690]
  [Iabc_grid] -> [Iabc_690]
  [fscan] -> Bus Creator1/19

== system SYHW_Zscan/SC_console/Fault Duration Select ==
  note: 20% - 0.625 sec
      | 35% - 0.92 sec
      | 50% - 1.214 sec
      | 75% - 1.705 sec
      | 90% - 2.0 sec
      | 130% - 0.5 sec
      | 125% - 1.0 sec
      | 120% - 10 sec
  1 : Constant  Value=0.625
  2 : Constant  Value=0.92
  3 : Constant  Value=1.214
  4 : Constant  Value=1.705
  5 : Constant  Value=2.0
  6 : Constant  Value=0.5
  7 : Constant
  8 : Constant  Value=10
  Multiport Switch : MultiPortSwitch  Inputs=8  DataPortForDefault=Additional data port
  index : Constant  Value=var_dur
  Out : Outport
  wires:
  6/1 -> Multiport Switch/7
  8/1 -> Multiport Switch/9
  7/1 -> Multiport Switch/8
  Multiport Switch/1 -> Out/1
  5/1 -> Multiport Switch/6
  4/1 -> Multiport Switch/5
  3/1 -> Multiport Switch/4
  2/1 -> Multiport Switch/3
  1/1 -> Multiport Switch/2, Multiport Switch/10
  index/1 -> Multiport Switch/1  "FaultDuration"

== system SYHW_Zscan/SC_console/扫频输入模块 ==
  Mux2 : Mux
  q10 : Constant  Value=DisRatio1
  q11 : Constant  Value=DisRatio2
  q12 : Constant  Value=ScanStart
  q8 : Constant  Value=fileNum
  scan : Outport
  wires:
  Mux2/1 -> scan/1
  q8/1 -> Mux2/4  "文件编号"
  q10/1 -> Mux2/2  "扰动百分比1"
  q11/1 -> Mux2/3  "扰动百分比2"
  q12/1 -> Mux2/1  "扫频触发"

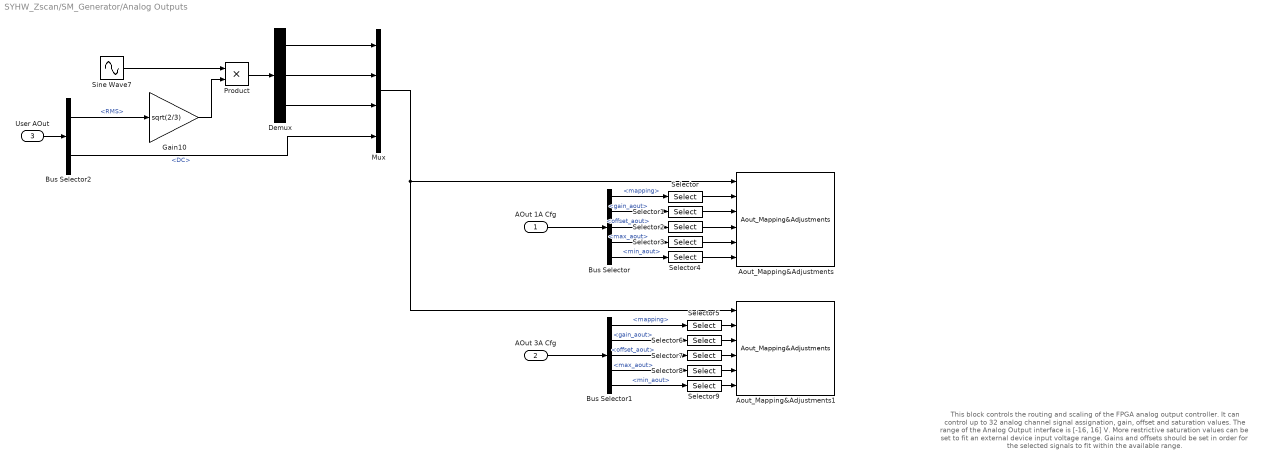
== system SYHW_Zscan/SM_Generator/Analog Outputs ==
  note: This block controls the routing and scaling of the FPGA analog
      | output controller.
      |
      |  It can control up to 32 analog channel signal assignation, gain,
      | offset and saturation values.
      |
      | The range of the Analog Output interface is [-16, 16] V.  More
      | restrictive saturation values can be set to fit an external device
      | input voltage range. Gains and offsets should be set in order for
      | the selected signals to fit within the available range.
  AOut 1A Cfg : Inport
  AOut 3A Cfg : Inport  Port=2
  User AOut : Inport  Port=3
  Aout_Mapping&Adjustments : cpuhilios_lib/Aout_Mapping&Adjustments  ChNum=16 (1 Aout mezz)  UserAoutNum=4  block_index=0  DataInId=15  LoadInId=4  CtrlerName='eHS Ctrl'
      settings: AttributesFormatString=%<CtrlerName>
  Aout_Mapping&Adjustments1 : cpuhilios_lib/Aout_Mapping&Adjustments  ChNum=16 (1 Aout mezz)  UserAoutNum=4  block_index=0  DataInId=21  LoadInId=22  CtrlerName='eHS Ctrl'
      settings: AttributesFormatString=%<CtrlerName>
  Bus Selector : BusSelector  OutputSignals=mapping,gain_aout,offset_aout,max_aout,min_aout
  Bus Selector1 : BusSelector  OutputSignals=mapping,gain_aout,offset_aout,max_aout,min_aout
  Bus Selector2 : BusSelector  OutputSignals=RMS,DC
  Demux : Demux  Outputs=3
  Gain10 : Gain  Gain=sqrt(2/3)
  Mux : Mux
  Product : Product
  Selector{,1..9} (10 alike) : Selector  InputPortWidth=32  IndexOptions=Index vector (dialog)  Indices=[1:1:16]  OutputSizes=1
  Sine Wave7 : Sin  Frequency=100*pi  Phase=[0 -2*pi/3 2*pi/3]  SampleTime=0
  wires:
  Bus Selector/2 -> Selector1/1  "<gain_aout>"
  Bus Selector/5 -> Selector4/1  "<min_aout>"
  Bus Selector/4 -> Selector3/1  "<max_aout>"
  Bus Selector/1 -> Selector/1  "<mapping>"
  Bus Selector/3 -> Selector2/1  "<offset_aout>"
  AOut 1A Cfg/1 -> Bus Selector/1
  Selector/1 -> Aout_Mapping&Adjustments/2
  Selector1/1 -> Aout_Mapping&Adjustments/3
  Selector2/1 -> Aout_Mapping&Adjustments/4
  Selector3/1 -> Aout_Mapping&Adjustments/5
  Selector4/1 -> Aout_Mapping&Adjustments/6
  Bus Selector1/2 -> Selector6/1  "<gain_aout>"
  Bus Selector1/5 -> Selector9/1  "<min_aout>"
  Bus Selector1/4 -> Selector8/1  "<max_aout>"
  Bus Selector1/1 -> Selector5/1  "<mapping>"
  Bus Selector1/3 -> Selector7/1  "<offset_aout>"
  Selector5/1 -> Aout_Mapping&Adjustments1/2
  Selector6/1 -> Aout_Mapping&Adjustments1/3
  Selector7/1 -> Aout_Mapping&Adjustments1/4
  Selector8/1 -> Aout_Mapping&Adjustments1/5
  Selector9/1 -> Aout_Mapping&Adjustments1/6
  AOut 3A Cfg/1 -> Bus Selector1/1
  Mux/1 -> Aout_Mapping&Adjustments1/1, Aout_Mapping&Adjustments/1
  User AOut/1 -> Bus Selector2/1
  Sine Wave7/1 -> Product/1
  Gain10/1 -> Product/2
  Bus Selector2/1 -> Gain10/1  "<RMS>"
  Product/1 -> Demux/1
  Demux/1 -> Mux/1
  Demux/2 -> Mux/2
  Demux/3 -> Mux/3
  Bus Selector2/2 -> Mux/4  "<DC>"

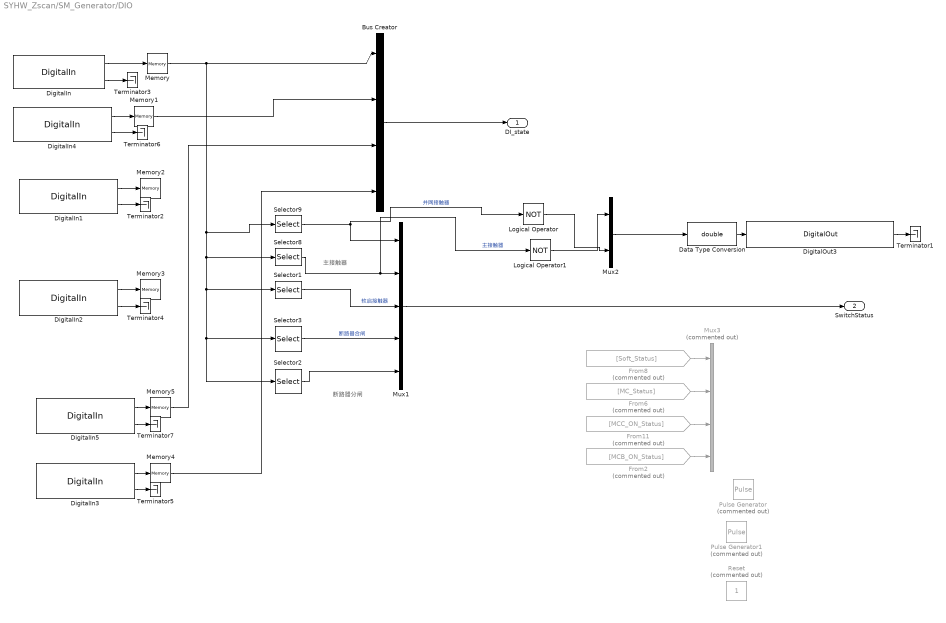
== system SYHW_Zscan/SM_Generator/DIO ==
  note: 断路器分闸
  note: 主接触器
  Bus Creator : BusCreator
  Data Type Conversion : DataTypeConversion  OutDataTypeStr=double
  DigitalIn : rtio_opalrt_common/DigitalIn  CtrlName='eHS Ctrl'  portNb=9  FcnNos=Slot 4 Module A Subsection 1  size=1  maxcount=8  count=8  sampleTime=0  numchan=8
      settings: AttributesFormatString=%<CtrlName>
  DigitalIn1 : rtio_opalrt_common/DigitalIn  CtrlName='eHS Ctrl'  portNb=11  FcnNos=Slot 4 Module A Subsection 3  size=1  maxcount=8  count=8  sampleTime=0  numchan=8
      settings: AttributesFormatString=%<CtrlName>
  DigitalIn2 : rtio_opalrt_common/DigitalIn  CtrlName='eHS Ctrl'  portNb=12  FcnNos=Slot 4 Module A Subsection 4  size=1  maxcount=8  count=8  sampleTime=0  numchan=8
      settings: AttributesFormatString=%<CtrlName>
  DigitalIn3 : rtio_opalrt_common/DigitalIn  CtrlName='eHS Ctrl'  portNb=6  FcnNos=Slot 2 Module A Subsection 2  size=1  maxcount=8  count=8  sampleTime=0  numchan=8
      settings: AttributesFormatString=%<CtrlName>
  DigitalIn4 : rtio_opalrt_common/DigitalIn  CtrlName='eHS Ctrl'  portNb=10  FcnNos=Slot 4 Module A Subsection 2  size=1  maxcount=8  count=8  sampleTime=0  numchan=8
      settings: AttributesFormatString=%<CtrlName>
  DigitalIn5 : rtio_opalrt_common/DigitalIn  CtrlName='eHS Ctrl'  portNb=5  FcnNos=Slot 2 Module A Subsection 1  size=1  maxcount=8  count=8  sampleTime=0  numchan=8
      settings: AttributesFormatString=%<CtrlName>
  DigitalOut3 : rtio_opalrt_common/DigitalOut  CtrlName='eHS Ctrl'  portNb=12  FcnNos=Slot 2 Module B Subsection 2  size=8  maxcount=8  count=2  numchan=2
      settings: AttributesFormatString=%<CtrlName>
  From11 : From  Commented=on  GotoTag=MCC_ON_Status
      settings: CloseFcn=tagdialog Close
  From2 : From  Commented=on  GotoTag=MCB_ON_Status
      settings: CloseFcn=tagdialog Close
  From6 : From  Commented=on  GotoTag=MC_Status
      settings: CloseFcn=tagdialog Close
  From8 : From  Commented=on  GotoTag=Soft_Status
      settings: CloseFcn=tagdialog Close
  Logical Operator : Logic  Operator=NOT  AllPortsSameDT=off
  Logical Operator1 : Logic  Operator=NOT  AllPortsSameDT=off
  Memory{,1..5} (6 alike) : Memory
  Mux1 : Mux  Inputs=5
  Mux2 : Mux  Inputs=2
  Mux3 : Mux  Commented=on
  Pulse Generator : DiscretePulseGenerator  Commented=on  PulseType=Time based  Period=1  PulseWidth=5
  Pulse Generator1 : DiscretePulseGenerator  Commented=on  PulseType=Time based  Period=1  PulseWidth=5
  Reset : Constant  Commented=on
  Selector1 : Selector  InputPortWidth=8  IndexOptions=Index vector (dialog)  Indices=[2]  OutputSizes=1
  Selector2 : Selector  InputPortWidth=8  IndexOptions=Index vector (dialog)  Indices=[5]  OutputSizes=1
  Selector3 : Selector  InputPortWidth=8  IndexOptions=Index vector (dialog)  Indices=[4]  OutputSizes=1
  Selector8 : Selector  InputPortWidth=8  IndexOptions=Index vector (dialog)  Indices=[1]  OutputSizes=1
  Selector9 : Selector  InputPortWidth=8  IndexOptions=Index vector (dialog)  Indices=[3]  OutputSizes=1
  Terminator{1..7} (7 alike) : Terminator
  DI_state : Outport
  SwitchStatus : Outport  Port=2
  wires:
  DigitalIn/2 -> Terminator3/1
  DigitalIn/1 -> Memory/1
  DigitalIn1/2 -> Terminator2/1
  DigitalIn4/1 -> Memory1/1
  DigitalIn4/2 -> Terminator6/1
  DigitalIn1/1 -> Memory2/1
  Memory1/1 -> Bus Creator/2
  DigitalOut3/1 -> Terminator1/1
  Mux1/1 -> SwitchStatus/1
  From8/1 -> Mux3/1
  From6/1 -> Mux3/2
  From11/1 -> Mux3/3
  From2/1 -> Mux3/4
  Selector9/1 -> Mux1/1, Logical Operator/1  "并网接触器"
  Selector8/1 -> Logical Operator1/1, Mux1/2  "主接触器"
  Selector1/1 -> Mux1/3  "软启接触器"
  Selector3/1 -> Mux1/4  "断路器合闸"
  Selector2/1 -> Mux1/5
  Bus Creator/1 -> DI_state/1
  Memory5/1 -> Bus Creator/3
  Memory/1 -> Selector8/1, Selector2/1, Selector3/1, Selector1/1, Selector9/1, Bus Creator/1
  Data Type Conversion/1 -> DigitalOut3/1
  Logical Operator/1 -> Mux2/2
  Logical Operator1/1 -> Mux2/1
  Mux2/1 -> Data Type Conversion/1
  DigitalIn2/2 -> Terminator4/1
  DigitalIn2/1 -> Memory3/1
  Memory4/1 -> Bus Creator/4
  DigitalIn3/2 -> Terminator5/1
  DigitalIn3/1 -> Memory4/1
  DigitalIn5/2 -> Terminator7/1
  DigitalIn5/1 -> Memory5/1

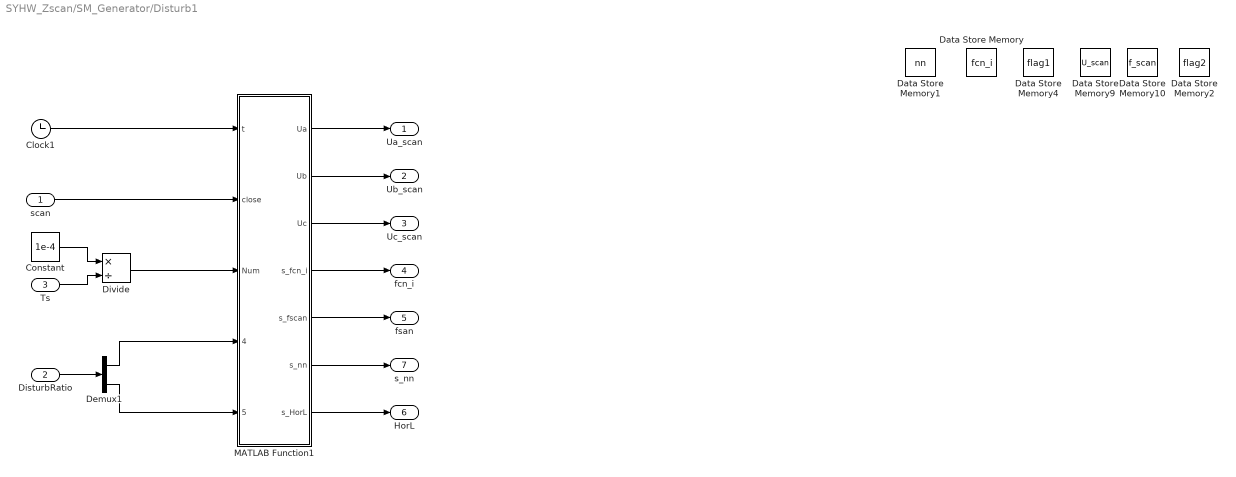
== system SYHW_Zscan/SM_Generator/Disturb1 ==
  scan : Inport
  DisturbRatio : Inport  Port=2
  Ts : Inport  Port=3
  Clock1 : Clock
  Constant : Constant  Value=1e-4
  Data Store Memory : DataStoreMemory  DataStoreName=fcn_i  ReadBeforeWriteMsg=warning  WriteAfterWriteMsg=warning  WriteAfterReadMsg=warning  OutDataTypeStr=double
  Data Store Memory1 : DataStoreMemory  DataStoreName=nn  ReadBeforeWriteMsg=warning  WriteAfterWriteMsg=warning  WriteAfterReadMsg=warning  OutDataTypeStr=double
  Data Store Memory10 : DataStoreMemory  DataStoreName=f_scan  ReadBeforeWriteMsg=warning  WriteAfterWriteMsg=warning  WriteAfterReadMsg=warning  OutDataTypeStr=double
  Data Store Memory2 : DataStoreMemory  DataStoreName=flag2  ReadBeforeWriteMsg=warning  WriteAfterWriteMsg=warning  WriteAfterReadMsg=warning  OutDataTypeStr=double
  Data Store Memory4 : DataStoreMemory  DataStoreName=flag1  ReadBeforeWriteMsg=warning  WriteAfterWriteMsg=warning  WriteAfterReadMsg=warning  OutDataTypeStr=double
  Data Store Memory9 : DataStoreMemory  DataStoreName=U_scan  ReadBeforeWriteMsg=warning  WriteAfterWriteMsg=warning  WriteAfterReadMsg=warning  OutDataTypeStr=double
  Demux1 : Demux  Outputs=2
  Divide : Product  Inputs=*/
  MATLAB Function1 : MATLAB Function  RequirementInfo={} %GIDa_fecc14f3_1c77_4fe4_adda_960a052a1091  TreatAsAtomicUnit=on  SystemSampleTime=Ts
  Ua_scan : Outport
  Ub_scan : Outport  Port=2
  Uc_scan : Outport  Port=3
  fcn_i : Outport  Port=4
  fsan : Outport  Port=5
  HorL : Outport  Port=6
  "s_nn " : Outport  Port=7
  wires:
  MATLAB Function1/6(s_nn) -> "s_nn "/1
  MATLAB Function1/5(s_fscan) -> fsan/1
  MATLAB Function1/7(s_HorL) -> HorL/1
  MATLAB Function1/4(s_fcn_i) -> fcn_i/1
  MATLAB Function1/3(Uc) -> Uc_scan/1
  MATLAB Function1/1(Ua) -> Ua_scan/1
  MATLAB Function1/2(Ub) -> Ub_scan/1
  Clock1/1 -> MATLAB Function1/1(t)
  DisturbRatio/1 -> Demux1/1
  Demux1/2 -> MATLAB Function1/5(ScanRatio2)
  Demux1/1 -> MATLAB Function1/4(ScanRatio1)
  Ts/1 -> Divide/2
  Constant/1 -> Divide/1
  Divide/1 -> MATLAB Function1/3(Num)
  scan/1 -> MATLAB Function1/2(close)
